simulink model "TDM_simulink"  (R2018a)
settings: Solver=ode45  StartTime=0.0  StopTime=10.0  RelTol=1e-3  EnableMultiTasking=on
libraries: dspsigops x4
settings Model: Creator=Abhilash  LastModifiedBy=ASUS
settings DataIOCC: LimitDataPoints=on  SaveFormat=Array  SignalLoggingSaveFormat=ModelDataLogs
settings OptimizationCC: ExpressionDepthLimit=2147483647  LifeSpan=inf
settings DebuggingCC: UnderspecifiedInitializationDetection=Classic  MergeDetectMultiDrivingBlocksExec=none  SolverPrmCheckMsg=warning  FcnCallInpInsideContextMsg=warning  StateNameClashWarn=warning  SFUnexpectedBacktrackingDiag=warning  SFNoUnconditionalDefaultTransitionDiag=warning  SFExecutionAtInitializationDiag=none
settings HardwareCC: ProdBitPerPointer=32  ProdBitPerSizeT=32  ProdBitPerPtrDiffT=32  ProdLargestAtomicFloat=None  ProdIntDivRoundTo=Undefined  ProdEndianess=Unspecified  ProdWordSize=32  ProdHWDeviceType=32-bit Generic
settings ModelReferenceCC: PropagateSignalLabelsOutOfModel=off
settings CodeAppCC: StateflowObjectComments=on
settings GRTTargetCC: TargetLangStandard=C89/C90 (ANSI)  CombineOutputUpdateFcns=off  GRTInterface=on
settings ConfigComp: CovMetricSettings=dw  CovHtmlReporting=on  CovSaveCumulativeToWorkspaceVar=on  CovSaveSingleToWorkspaceVar=on  CovExternalEMLEnable=off

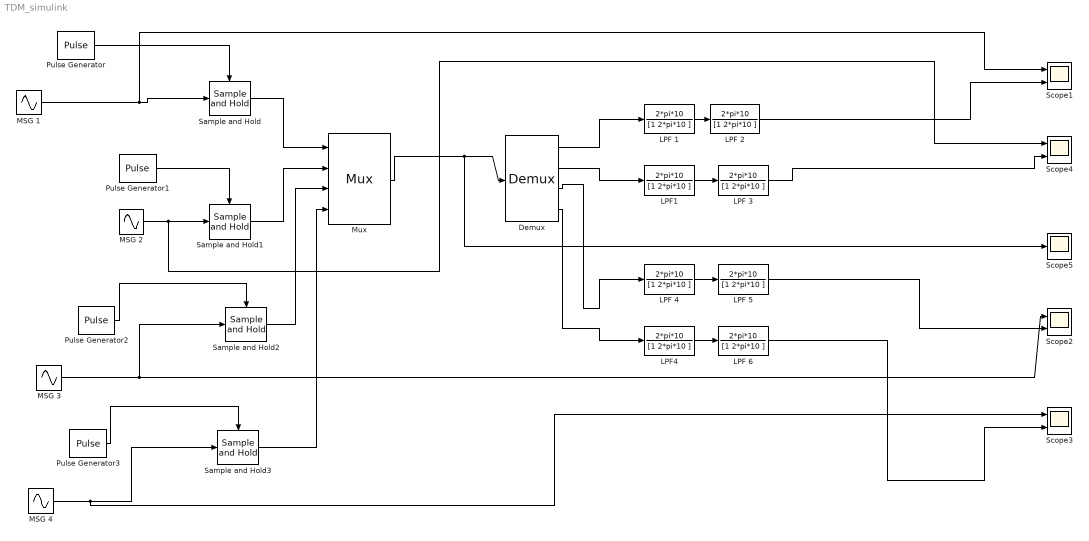
== system TDM_simulink ==
  Demux : Demux
  LPF {1..6} (6 alike) : TransferFcn  Numerator=2*pi*10  Denominator=[1 2*pi*10 ]
  LPF1 : TransferFcn  Numerator=2*pi*10  Denominator=[1 2*pi*10 ]
  LPF4 : TransferFcn  Numerator=2*pi*10  Denominator=[1 2*pi*10 ]
  MSG 1 : Sin  Frequency=2  SampleTime=0
  MSG 2 : Sin  Frequency=4  SampleTime=0
  MSG 3 : Sin  Frequency=6  SampleTime=0
  MSG 4 : Sin  Frequency=8  SampleTime=0
  Mux : Mux
  Pulse Generator{,1..3} (4 alike) : DiscretePulseGenerator  PulseType=Time based  Period=.01  PulseWidth=5
  Sample and Hold{,1..3} (4 alike) : dspsigops/Sample and Hold  trig=Rising edge  initCond=0  latchinput=off
  Scope{1..4} (4 alike) : Scope  NumInputPorts=2
  Scope5 : Scope
  wires:
  Pulse Generator/1 -> Sample and Hold/Trigger
  MSG 1/1 -> Scope1/1, Sample and Hold/1
  Pulse Generator1/1 -> Sample and Hold1/Trigger
  MSG 2/1 -> Scope4/1, Sample and Hold1/1
  Sample and Hold/1 -> Mux/1
  Mux/1 -> Scope5/1, Demux/1
  Demux/2 -> LPF1/1
  Demux/1 -> LPF 1/1
  Sample and Hold1/1 -> Mux/2
  LPF 1/1 -> LPF 2/1
  LPF1/1 -> LPF 3/1
  Pulse Generator2/1 -> Sample and Hold2/Trigger
  MSG 3/1 -> Sample and Hold2/1, Scope2/1
  Sample and Hold2/1 -> Mux/3
  Pulse Generator3/1 -> Sample and Hold3/Trigger
  MSG 4/1 -> Scope3/1, Sample and Hold3/1
  Sample and Hold3/1 -> Mux/4
  Demux/4 -> LPF4/1
  Demux/3 -> LPF 4/1
  LPF 4/1 -> LPF 5/1
  LPF4/1 -> LPF 6/1
  LPF 2/1 -> Scope1/2
  LPF 5/1 -> Scope2/2
  LPF 6/1 -> Scope3/2
  LPF 3/1 -> Scope4/2
